simulink model "motor"  (R2016a)
settings: Solver=VariableStepAuto  StartTime=0.0  StopTime=10.0  RelTol=1e-3
undefined symbols (not defined in the file or in its folder): b, J, lambdam, Ld, Lq, P, Rs, Vd, Vq
settings Model: Creator=jesse  LastModifiedBy=jesse

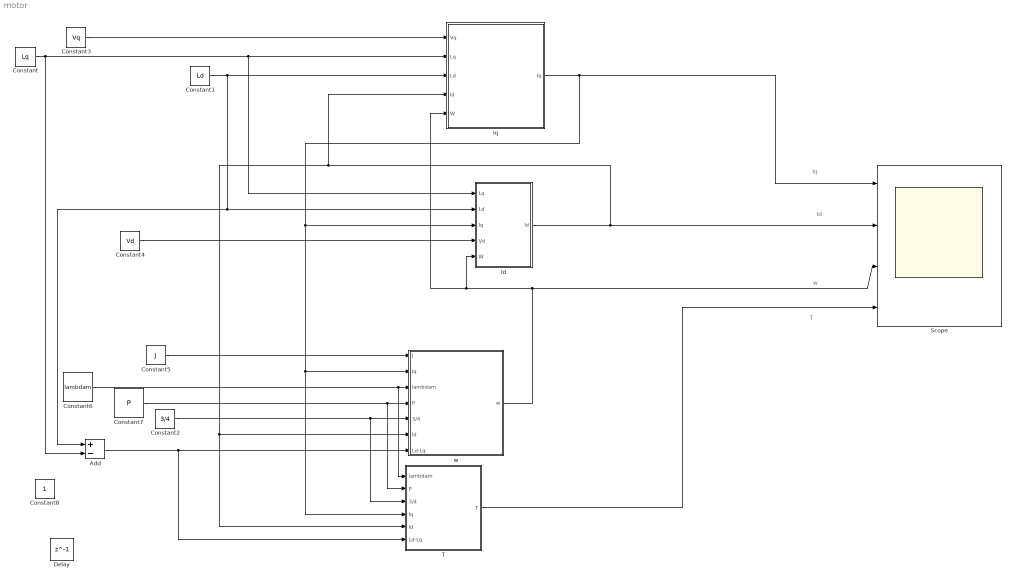
== system motor ==
  note: T
  note: w
  note: Id
  note: Iq
  Add : Sum  Inputs=+-
  Constant : Constant  Value=Lq
  Constant1 : Constant  Value=Ld
  Constant2 : Constant  Value=3/4
  Constant3 : Constant  Value=Vq
  Constant4 : Constant  Value=Vd
  Constant5 : Constant  Value=J
  Constant6 : Constant  Value=lambdam
  Constant7 : Constant  Value=P
  Constant8 : Constant
  Delay : Delay  DelayLength=1  InitialCondition=0
  Id : Subsystem
  Iq : Subsystem
  Scope : Scope  NumInputPorts=4
  T : Subsystem
  w : Subsystem
  wires:
  Constant/1 -> Add/2, Id/1("Lq "), Iq/2(Lq)
  Constant2/1 -> w/5("3/4 "), T/3(3/4)
  Constant6/1 -> T/1(lambdam), w/3(lambdam)
  Constant7/1 -> T/2(P), w/4(P)
  Add/1 -> T/6(Ld-Lq), w/7(Ld-Lq)
  Constant1/1 -> Id/2(Ld), Add/1, Iq/3(Ld)
  T/1(T) -> Scope/4
  w/1(w) -> Scope/3, Iq/5(W), Id/5(W)
  Constant5/1 -> w/1(J)
  Id/1(Id) -> Iq/4(Id), w/6(Id), T/5(Id), Scope/2
  Constant4/1 -> Id/4(Vd)
  Iq/1(Iq) -> Id/3(Iq), T/4(Iq), w/2(Iq), Scope/1
  Constant3/1 -> Iq/1(Vq)

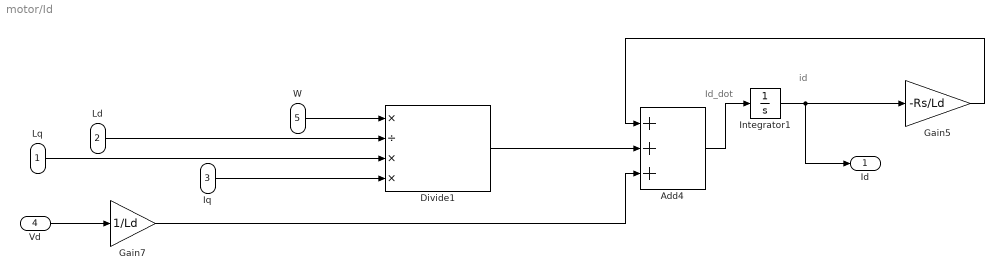
== system motor/Id ==
  note: Id_dot
  note: id
  "Lq " : Inport
  Ld : Inport  Port=2
  Iq : Inport  Port=3
  Vd : Inport  Port=4
  W : Inport  Port=5
  Add4 : Sum  Inputs=+++
  Divide1 : Product  Inputs=*/**
  Gain5 : Gain  Gain=-Rs/Ld
  Gain7 : Gain  Gain=1/Ld
  Integrator1 : Integrator
  Id : Outport
  wires:
  Ld/1 -> Divide1/2
  "Lq "/1 -> Divide1/3
  W/1 -> Divide1/1
  Gain7/1 -> Add4/3
  Add4/1 -> Integrator1/1
  Divide1/1 -> Add4/2
  Gain5/1 -> Add4/1
  Vd/1 -> Gain7/1
  Integrator1/1 -> Id/1, Gain5/1
  Iq/1 -> Divide1/4

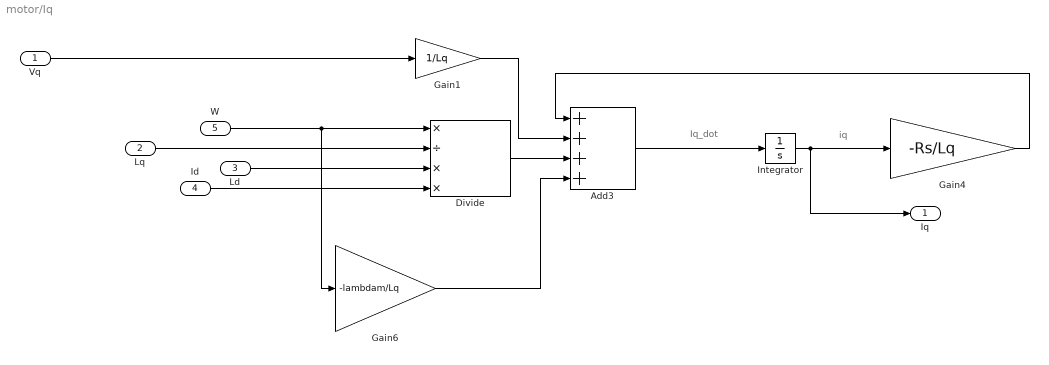
== system motor/Iq ==
  note: Iq_dot
  note: iq
  Vq : Inport
  Lq : Inport  Port=2
  Ld : Inport  Port=3
  Id : Inport  Port=4
  W : Inport  Port=5
  Add3 : Sum  Inputs=++++
  Divide : Product  Inputs=*/**
  Gain1 : Gain  Gain=1/Lq
  Gain4 : Gain  Gain=-Rs/Lq
  Gain6 : Gain  Gain=-lambdam/Lq
  Integrator : Integrator
  Iq : Outport
  wires:
  W/1 -> Gain6/1, Divide/1
  Integrator/1 -> Gain4/1, Iq/1
  Id/1 -> Divide/4
  Lq/1 -> Divide/2
  Ld/1 -> Divide/3
  Gain4/1 -> Add3/1
  Add3/1 -> Integrator/1
  Divide/1 -> Add3/3
  Gain1/1 -> Add3/2
  Vq/1 -> Gain1/1
  Gain6/1 -> Add3/4

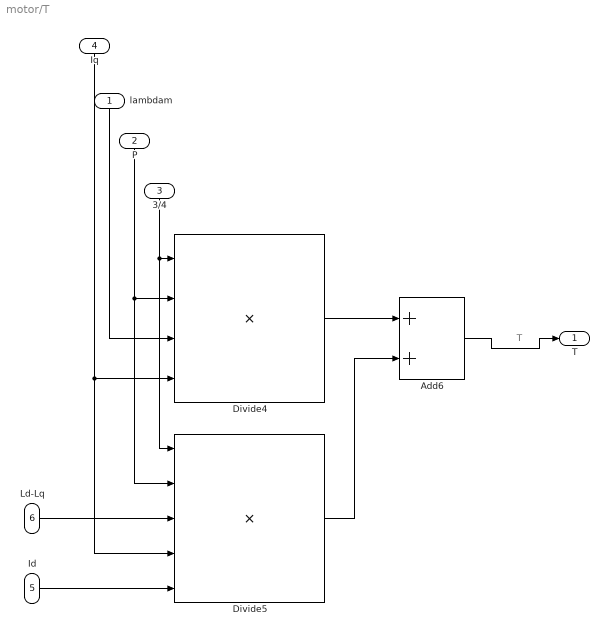
== system motor/T ==
  note: T
  lambdam : Inport
  P : Inport  Port=2
  3/4 : Inport  Port=3
  Iq : Inport  Port=4
  Id : Inport  Port=5
  Ld-Lq : Inport  Port=6
  Add6 : Sum
  Divide4 : Product  Inputs=****
  Divide5 : Product  Inputs=*****
  T : Outport
  wires:
  Divide5/1 -> Add6/2
  Divide4/1 -> Add6/1
  Add6/1 -> T/1
  Id/1 -> Divide5/5
  P/1 -> Divide5/2, Divide4/2
  Ld-Lq/1 -> Divide5/3
  Iq/1 -> Divide4/4, Divide5/4
  3/4/1 -> Divide5/1, Divide4/1
  lambdam/1 -> Divide4/3

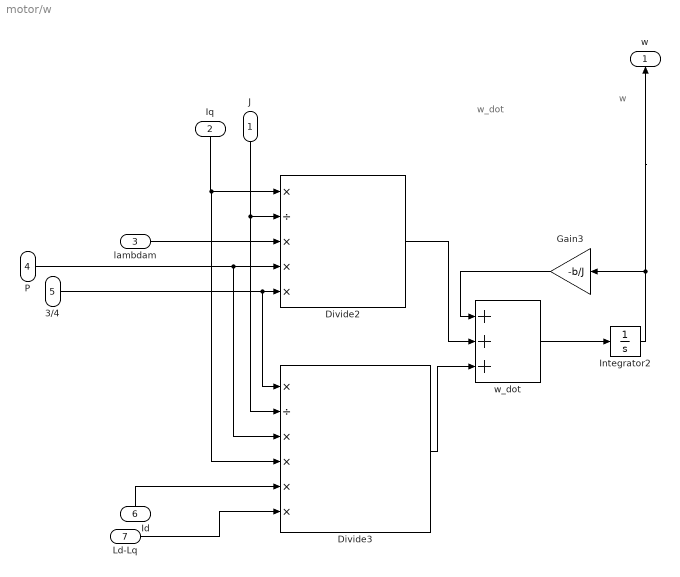
== system motor/w ==
  note: w_dot
  note: w
  J : Inport
  Iq : Inport  Port=2
  lambdam : Inport  Port=3
  P : Inport  Port=4
  "3/4 " : Inport  Port=5
  Id : Inport  Port=6
  Ld-Lq : Inport  Port=7
  Divide2 : Product  Inputs=*/***
  Divide3 : Product  Inputs=*/****
  Gain3 : Gain  Gain=-b/J
  Integrator2 : Integrator
  w_dot : Sum  Inputs=+++
  w : Outport
  wires:
  Id/1 -> Divide3/5
  Iq/1 -> Divide2/1, Divide3/4
  P/1 -> Divide3/3, Divide2/4
  lambdam/1 -> Divide2/3
  Integrator2/1 -> w/1, Gain3/1
  "3/4 "/1 -> Divide3/1, Divide2/5
  Ld-Lq/1 -> Divide3/6
  J/1 -> Divide3/2, Divide2/2
  Divide2/1 -> w_dot/2
  w_dot/1 -> Integrator2/1
  Divide3/1 -> w_dot/3
  Gain3/1 -> w_dot/1
